simulink model "test_ref_model"  (R2020a)
settings: Solver=FixedStepDiscrete  StartTime=0.0  StopTime=10.0  FixedStep=0.01  RelTol=1e-3
model mask{a=a, b=b}
model workspace (MAT data in the model file):
  a = 0
  b = 0
settings Model: ParameterArgumentNames=a,b  OrderedModelArguments=off  Creator=1014721  LastModifiedBy=1014721
settings OptimizationCC: DefaultParameterBehavior=Inlined  EnhancedBackFolding=on  PassReuseOutputArgsAs=Individual arguments  ZeroExternalMemoryAtStartup=off  ZeroInternalMemoryAtStartup=off  OptimizeBlockOrder=speed  DifferentSizesBufferReuse=on  OptimizationCustomize=off  EfficientTunableParamExpr=on
settings DebuggingCC: ParameterTunabilityLossMsg=error
settings SFSimCC: MATLABDynamicMemAlloc=off
settings RTWCC: SystemTargetFile=ert.tlc  GenCodeOnly=on  TemplateMakefile=ert_default_tmf
settings CodeAppCC: ForceParamTrailComments=on  IgnoreCustomStorageClasses=off  OperatorAnnotations=on  SimulinkDataObjDesc=on  SFDataObjDesc=on  InsertBlockDesc=on
settings ERTTargetCC: TargetLangStandard=C99 (ISO)  GenerateSampleERTMain=on  InlinedParameterPlacement=NonHierarchical  ERTCustomFileTemplate=example_file_process.tlc

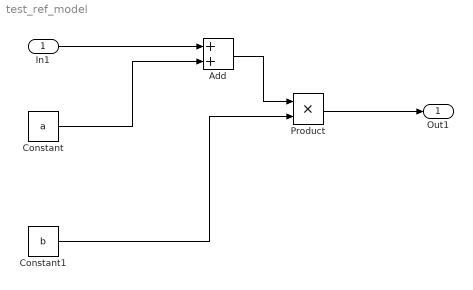
== system test_ref_model ==
  In1 : Inport  OutDataTypeStr=int32
  Add : Sum
  Constant : Constant  Value=a  OutDataTypeStr=int32
  Constant1 : Constant  Value=b  OutDataTypeStr=int32
  Product : Product  OutDataTypeStr=int32
  Out1 : Outport  OutDataTypeStr=int32
  wires:
  Constant/1 -> Add/2
  In1/1 -> Add/1
  Add/1 -> Product/1
  Constant1/1 -> Product/2
  Product/1 -> Out1/1
